simulink model "bh_SIM_7dof_car_VALIDATE"  (R2021a)
settings: Solver=ode15s  StartTime=0.0  StopTime=60  FixedStep=0.0005  RelTol=1e-5
libraries: simulink x1
settings Model: Creator=bhorton  LastModifiedBy=bhorton
settings SolverCC: ZeroCrossAlgorithm=Adaptive
settings ExplorerConfigSet: InternalSimMechanicsExplorerSettings="<ExplorerConfiguration><canonicalview>default</canonicalview><AnimationSetting><BasePlaybackSpeed>1.0</BasePlaybackSpeed><PlaybackSpeedFactor>1.0</PlaybackSpeedFactor></AnimationSetting><TilePanel><TileInfo><Tiles Columns=\"2\" Count=\"3\" Rows=\"2\"><Column Weight=\"0.4994\"/><Column Weight=\"0.5006\"/><Row Weight=\"0.4993\"/><Row Weight=\"0.5007\"/><Tile Height=\"1\" Width=\"2\" X=\"0\" Y=\"0\"/><Tile Height=\"1\" Width=\"1\" X=\"0\" Y=\"1\"/><Tile Height=\"1\" Width=\"1\" X=\"1\" Y=\"1\"/></Tiles></TileInfo><SceneInfo><SceneViewer><BGColor><R>0.60000002384185791</R><G>0.60000002384185791</G><B>0.60000002384185791</B></BGColor><Camera><DoPerspective>off</DoPerspective><Position><X>4.58629206826182401</X><Y>2.2090645401570459</Y><Z>2.36549759190957332</Z></Position><Center><X>2.57683900679416</X><Y>1.27770136551759128</Y><Z>-0.515230289296268573</Z></Center><Up><X>-0.185673330126828295</X><Y>0.96548958646651295</Y><Z>-0.182634259941381938</Z></Up><ViewLimDist>1</ViewLimDist><YLim>2.38220316698246792</YLim><XLim>4.86337026375055714</XLim></Camera></SceneViewer><SceneViewer><BGColor><R>0.60000002384185791</R><G>0.60000002384185791</G><B>0.60000002384185791</B></BGColor><Camera><DoPerspective>off</DoPerspective><Position><X>1.59253986433018846</X><Y>1.4781034625054259</Y><Z>2.45336125750569334</Z></Position><Center><X>1.41562813270534282</X><Y>1.03964723052633357</Y><Z>-0.792996094118513462</Z></Center><Up><X>-0.0228131350943184333</X><Y>0.990908416802929626</Y><Z>-0.132589857742894418</Z></Up><ViewLimDist>1</ViewLimDist><YLim>1.71081238252217549</YLim><XLim>1.71587395761839479</XLim></Camera></SceneViewer><SceneViewer><BGColor><R>0.60000002384185791</R><G>0.60000002384185791</G><B>0.60000002384185791</B></BGColor><Camera><DoPerspective>off</DoPerspective><Position><X>5.22556337212071131</X><Y>1.49802244333944778</Y><Z>-0.435936726178495881</Z></Position><Center><X>1.55561505094653896</X><Y>1.09424096945505833</Y><Z>-0.658674871233751014</Z></Center><Up><X>-0.109797444713875203</X><Y>0.993927323497863835</Y><Z>0.0072798858972461869</Z></Up><ViewLimDist>1</ViewLimDist><YLim>2.32163445502303123</YLim><XLim>2.33537193700541623</XLim></Camera></SceneViewer></SceneInfo></TilePanel><MechEditorPanel><Cameras/><GfxPanelCameraMap/><VideoCreator><PlaybackSpeedRatio>1.0</PlaybackSpeedRatio><FrameRate>30</FrameRate><VideoFormat>MPEG-4</VideoFormat><FrameSize>[800 600]</FrameSize></VideoCreator></MechEditorPanel></ExplorerConfiguration>"

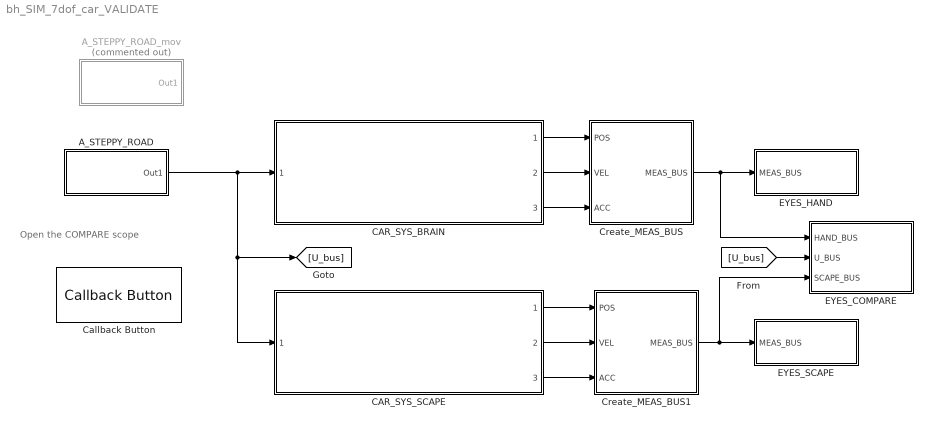
== system bh_SIM_7dof_car_VALIDATE ==
  note: Open the COMPARE scope
  A_STEPPY_ROAD : Subsystem
  A_STEPPY_ROAD_mov : Subsystem  Commented=on
  CAR_SYS_BRAIN : Subsystem  ReferencedSubsystem=bh_COMPONENT_model_7dof_car_HAND  L_b=OBJ_car_params.L_b  L_f=OBJ_car_params.L_f  L_R=OBJ_car_params.L_R  L_L=OBJ_car_params.L_L  m_c=OBJ_car_params.m_c  I_cZ=OBJ_car_params.I_cZ  I_cX=OBJ_car_params.I_cX  m_bR=OBJ_car_params.m_bR  m_fR=OBJ_car_params.m_fR  m_bL=OBJ_car_params.m_bL  m_fL=OBJ_car_params.m_fL  k_bR=OBJ_car_params.k_bR  k_fR=OBJ_car_params.k_fR  k_bL=OBJ_car_params.k_bL  k_fL=OBJ_car_params.k_fL  k_bRG=OBJ_car_params.k_bRG  k_fRG=OBJ_car_params.k_fRG  k_bLG=OBJ_car_params.k_bLG  k_fLG=OBJ_car_params.k_fLG  c_bR=OBJ_car_params.c_bR  c_fR=OBJ_car_params.c_fR  c_bL=OBJ_car_params.c_bL  c_fL=OBJ_car_params.c_fL  c_bRG=OBJ_car_params.c_bRG  c_fRG=OBJ_car_params.c_fRG  c_bLG=OBJ_car_params.c_bLG  c_fLG=OBJ_car_params.c_fLG  IC_pos=OBJ_car_params.IC_pos  IC_vel=OBJ_car_params.IC_vel
  CAR_SYS_SCAPE : Subsystem  ReferencedSubsystem=bh_COMPONENT_model_7dof_car_SCAPE  L_b=OBJ_car_params.L_b  L_f=OBJ_car_params.L_f  L_R=OBJ_car_params.L_R  L_L=OBJ_car_params.L_L  m_c=OBJ_car_params.m_c  I_cZ=OBJ_car_params.I_cZ  I_cX=OBJ_car_params.I_cX  m_bR=OBJ_car_params.m_bR  m_fR=OBJ_car_params.m_fR  m_bL=OBJ_car_params.m_bL  m_fL=OBJ_car_params.m_fL  k_bR=OBJ_car_params.k_bR  k_fR=OBJ_car_params.k_fR  k_bL=OBJ_car_params.k_bL  k_fL=OBJ_car_params.k_fL  k_bRG=OBJ_car_params.k_bRG  k_fRG=OBJ_car_params.k_fRG  k_bLG=OBJ_car_params.k_bLG  k_fLG=OBJ_car_params.k_fLG  c_bR=OBJ_car_params.c_bR  c_fR=OBJ_car_params.c_fR  c_bL=OBJ_car_params.c_bL  c_fL=OBJ_car_params.c_fL  c_bRG=OBJ_car_params.c_bRG  c_fRG=OBJ_car_params.c_fRG  c_bLG=OBJ_car_params.c_bLG  c_fLG=OBJ_car_params.c_fLG  IC_pos=OBJ_car_params.IC_pos  IC_vel=OBJ_car_params.IC_vel
  Callback Button : CallbackButton  ButtonText=CLICK me to open SCOPE
      settings: ClickFcn=open_system([bdroot,'/EYES_COMPARE/COMPARE_POS'])
  Create_MEAS_BUS : Subsystem
  Create_MEAS_BUS1 : Subsystem
  EYES_COMPARE : Subsystem
  EYES_HAND : Subsystem
  EYES_SCAPE : Subsystem
  wires:
  CAR_SYS_BRAIN/1 -> Create_MEAS_BUS/1(POS)
  CAR_SYS_BRAIN/2 -> Create_MEAS_BUS/2(VEL)
  CAR_SYS_BRAIN/3 -> Create_MEAS_BUS/3(ACC)
  Create_MEAS_BUS/1(MEAS_BUS) -> EYES_COMPARE/1(HAND_BUS), EYES_HAND/1(MEAS_BUS)
  CAR_SYS_SCAPE/1 -> Create_MEAS_BUS1/1(POS)
  CAR_SYS_SCAPE/2 -> Create_MEAS_BUS1/2(VEL)
  CAR_SYS_SCAPE/3 -> Create_MEAS_BUS1/3(ACC)
  Create_MEAS_BUS1/1(MEAS_BUS) -> EYES_COMPARE/3(SCAPE_BUS), EYES_SCAPE/1(MEAS_BUS)
  A_STEPPY_ROAD/1(Out1) -> [U_bus], CAR_SYS_SCAPE/1, CAR_SYS_BRAIN/1
  [U_bus] -> EYES_COMPARE/2(U_BUS)

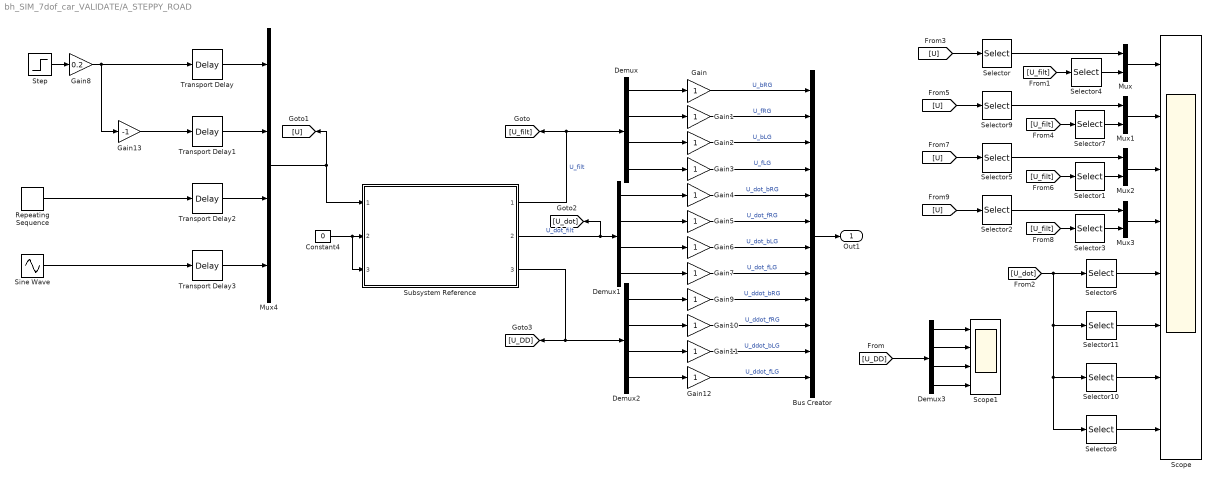
== system bh_SIM_7dof_car_VALIDATE/A_STEPPY_ROAD ==
  Bus Creator : BusCreator  Inputs=12
  Constant4 : Constant  Value=0
  Demux{,1..3} (4 alike) : Demux
  Gain{,1..7,9..12} (12 alike) : Gain
  Gain13 : Gain  Gain=-1
  Gain8 : Gain  Gain=0.2
  Mux{,1..3} (4 alike) : Mux  Inputs=2
  Mux4 : Mux
  Repeating Sequence : simulink/Sources/Repeating Sequence  rep_seq_t=[0 2]  rep_seq_y=[0 0.2]
  Scope : Scope  NumInputPorts=8
  Scope1 : Scope  NumInputPorts=4
  Selector : Selector  InputPortWidth=4  IndexOptions=Index vector (dialog)  Indices=1  OutputSizes=1
  Selector1 : Selector  InputPortWidth=4  IndexOptions=Index vector (dialog)  Indices=3  OutputSizes=1
  Selector10 : Selector  InputPortWidth=4  IndexOptions=Index vector (dialog)  Indices=3  OutputSizes=1
  Selector11 : Selector  InputPortWidth=4  IndexOptions=Index vector (dialog)  Indices=2  OutputSizes=1
  Selector2 : Selector  InputPortWidth=4  IndexOptions=Index vector (dialog)  Indices=4  OutputSizes=1
  Selector3 : Selector  InputPortWidth=4  IndexOptions=Index vector (dialog)  Indices=4  OutputSizes=1
  Selector4 : Selector  InputPortWidth=4  IndexOptions=Index vector (dialog)  Indices=1  OutputSizes=1
  Selector5 : Selector  InputPortWidth=4  IndexOptions=Index vector (dialog)  Indices=3  OutputSizes=1
  Selector6 : Selector  InputPortWidth=4  IndexOptions=Index vector (dialog)  Indices=1  OutputSizes=1
  Selector7 : Selector  InputPortWidth=4  IndexOptions=Index vector (dialog)  Indices=2  OutputSizes=1
  Selector8 : Selector  InputPortWidth=4  IndexOptions=Index vector (dialog)  Indices=4  OutputSizes=1
  Selector9 : Selector  InputPortWidth=4  IndexOptions=Index vector (dialog)  Indices=2  OutputSizes=1
  Sine Wave : Sin  Amplitude=0.25  Frequency=2*pi*3  SampleTime=0
  Step : Step  Time=0  SampleTime=0
  Subsystem Reference : Subsystem  ReferencedSubsystem=bh_COMPONENT_deriv_est  wn=2*pi*5000  p=1
  Transport Delay : TransportDelay  DelayTime=20
      settings: AttributesFormatString=Delay =%<DelayTime> (secs)
  Transport Delay1 : TransportDelay  DelayTime=30
      settings: AttributesFormatString=Delay =%<DelayTime> (secs)
  Transport Delay2 : TransportDelay  DelayTime=40
      settings: AttributesFormatString=Delay =%<DelayTime> (secs)
  Transport Delay3 : TransportDelay  DelayTime=50
      settings: AttributesFormatString=Delay =%<DelayTime> (secs)
  Out1 : Outport
  wires:
  Selector8/1 -> Scope/8
  Subsystem Reference/3 -> [U_DD], Demux2/1
  Demux2/4 -> Gain12/1
  Demux/3 -> Gain2/1
  Selector1/1 -> Mux2/2
  Gain5/1 -> Bus Creator/6  "U_dot_fRG"
  Subsystem Reference/1 -> [U_filt], Demux/1  "U_filt"
  Gain6/1 -> Bus Creator/7  "U_dot_bLG"
  Gain7/1 -> Bus Creator/8  "U_dot_fLG"
  Gain11/1 -> Bus Creator/11  "U_ddot_bLG"
  Subsystem Reference/2 -> [U_dot], Demux1/1  "U_dot_filt"
  Constant4/1 -> Subsystem Reference/3, Subsystem Reference/2
  [U_DD] -> Demux3/1
  Demux3/3 -> Scope1/3
  Demux3/2 -> Scope1/2
  Gain/1 -> Bus Creator/1  "U_bRG"
  Demux2/2 -> Gain10/1
  Selector2/1 -> Mux3/1
  Gain12/1 -> Bus Creator/12  "U_ddot_fLG"
  Gain9/1 -> Bus Creator/9  "U_ddot_bRG"
  Gain10/1 -> Bus Creator/10  "U_ddot_fRG"
  Mux1/1 -> Scope/2
  [U_filt] -> Selector3/1
  Selector6/1 -> Scope/5
  Demux3/4 -> Scope1/4
  Selector5/1 -> Mux2/1
  Demux2/3 -> Gain11/1
  Demux2/1 -> Gain9/1
  Mux2/1 -> Scope/3
  Demux3/1 -> Scope1/1
  Selector/1 -> Mux/1
  [U] -> Selector2/1
  Bus Creator/1 -> Out1/1
  Selector3/1 -> Mux3/2
  Selector7/1 -> Mux1/2
  Demux1/4 -> Gain7/1
  [U] -> Selector9/1
  Selector9/1 -> Mux1/1
  Mux3/1 -> Scope/4
  [U] -> Selector/1
  Selector4/1 -> Mux/2
  Mux/1 -> Scope/1
  [U_filt] -> Selector1/1
  [U] -> Selector5/1
  Demux1/3 -> Gain6/1
  Demux/2 -> Gain1/1
  [U_dot] -> Selector11/1, Selector10/1, Selector8/1, Selector6/1
  Demux/1 -> Gain/1
  Gain4/1 -> Bus Creator/5  "U_dot_bRG"
  [U_filt] -> Selector7/1
  [U_filt] -> Selector4/1
  Demux1/2 -> Gain5/1
  Gain3/1 -> Bus Creator/4  "U_fLG"
  Selector10/1 -> Scope/7
  Selector11/1 -> Scope/6
  Demux/4 -> Gain3/1
  Gain1/1 -> Bus Creator/2  "U_fRG"
  Demux1/1 -> Gain4/1
  Gain2/1 -> Bus Creator/3  "U_bLG"
  Mux4/1 -> Subsystem Reference/1, [U]
  Step/1 -> Gain8/1
  Transport Delay/1 -> Mux4/1
  Transport Delay1/1 -> Mux4/2
  Transport Delay2/1 -> Mux4/3
  Transport Delay3/1 -> Mux4/4
  Gain8/1 -> Gain13/1, Transport Delay/1
  Sine Wave/1 -> Transport Delay3/1
  Gain13/1 -> Transport Delay1/1
  Repeating Sequence/1 -> Transport Delay2/1

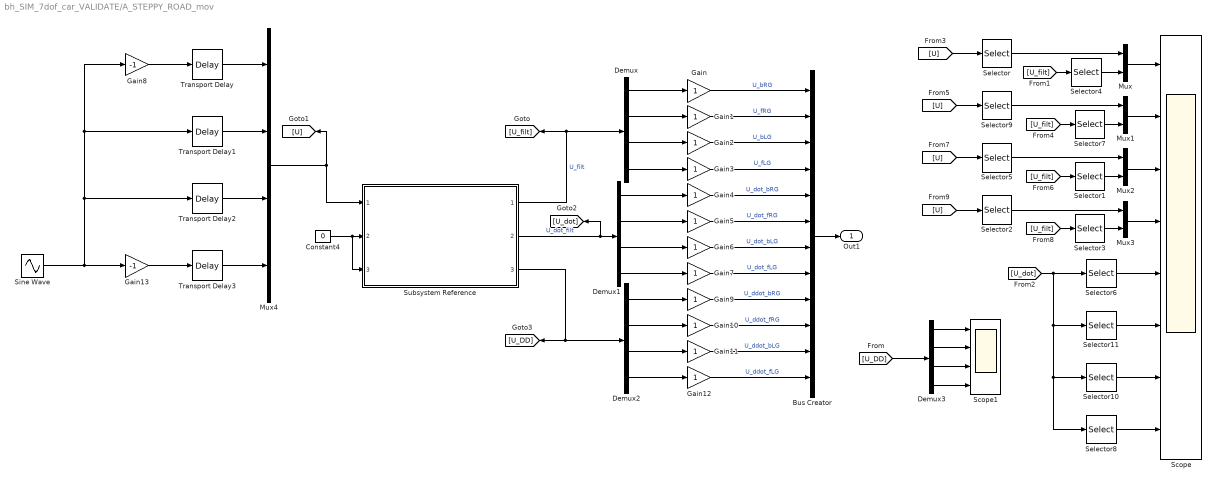
== system bh_SIM_7dof_car_VALIDATE/A_STEPPY_ROAD_mov ==
  Bus Creator : BusCreator  Inputs=12
  Constant4 : Constant  Value=0
  Demux{,1..3} (4 alike) : Demux
  Gain{,1..7,9..12} (12 alike) : Gain
  Gain13 : Gain  Gain=-1
  Gain8 : Gain  Gain=-1
  Mux{,1..3} (4 alike) : Mux  Inputs=2
  Mux4 : Mux
  Scope : Scope  NumInputPorts=8
  Scope1 : Scope  NumInputPorts=4
  Selector : Selector  InputPortWidth=4  IndexOptions=Index vector (dialog)  Indices=1  OutputSizes=1
  Selector1 : Selector  InputPortWidth=4  IndexOptions=Index vector (dialog)  Indices=3  OutputSizes=1
  Selector10 : Selector  InputPortWidth=4  IndexOptions=Index vector (dialog)  Indices=3  OutputSizes=1
  Selector11 : Selector  InputPortWidth=4  IndexOptions=Index vector (dialog)  Indices=2  OutputSizes=1
  Selector2 : Selector  InputPortWidth=4  IndexOptions=Index vector (dialog)  Indices=4  OutputSizes=1
  Selector3 : Selector  InputPortWidth=4  IndexOptions=Index vector (dialog)  Indices=4  OutputSizes=1
  Selector4 : Selector  InputPortWidth=4  IndexOptions=Index vector (dialog)  Indices=1  OutputSizes=1
  Selector5 : Selector  InputPortWidth=4  IndexOptions=Index vector (dialog)  Indices=3  OutputSizes=1
  Selector6 : Selector  InputPortWidth=4  IndexOptions=Index vector (dialog)  Indices=1  OutputSizes=1
  Selector7 : Selector  InputPortWidth=4  IndexOptions=Index vector (dialog)  Indices=2  OutputSizes=1
  Selector8 : Selector  InputPortWidth=4  IndexOptions=Index vector (dialog)  Indices=4  OutputSizes=1
  Selector9 : Selector  InputPortWidth=4  IndexOptions=Index vector (dialog)  Indices=2  OutputSizes=1
  Sine Wave : Sin  Amplitude=0.15  Frequency=2*pi*2  SampleTime=0
  Subsystem Reference : Subsystem  ReferencedSubsystem=bh_COMPONENT_deriv_est  wn=2*pi*5000  p=1
  Transport Delay{,1..3} (4 alike) : TransportDelay  DelayTime=10
      settings: AttributesFormatString=Delay =%<DelayTime> (secs)
  Out1 : Outport
  wires:
  Selector8/1 -> Scope/8
  Subsystem Reference/3 -> [U_DD], Demux2/1
  Demux2/4 -> Gain12/1
  Demux/3 -> Gain2/1
  Selector1/1 -> Mux2/2
  Gain5/1 -> Bus Creator/6  "U_dot_fRG"
  Subsystem Reference/1 -> [U_filt], Demux/1  "U_filt"
  Gain6/1 -> Bus Creator/7  "U_dot_bLG"
  Gain7/1 -> Bus Creator/8  "U_dot_fLG"
  Gain11/1 -> Bus Creator/11  "U_ddot_bLG"
  Subsystem Reference/2 -> [U_dot], Demux1/1  "U_dot_filt"
  Constant4/1 -> Subsystem Reference/3, Subsystem Reference/2
  [U_DD] -> Demux3/1
  Demux3/3 -> Scope1/3
  Demux3/2 -> Scope1/2
  Gain/1 -> Bus Creator/1  "U_bRG"
  Demux2/2 -> Gain10/1
  Selector2/1 -> Mux3/1
  Gain12/1 -> Bus Creator/12  "U_ddot_fLG"
  Gain9/1 -> Bus Creator/9  "U_ddot_bRG"
  Gain10/1 -> Bus Creator/10  "U_ddot_fRG"
  Mux1/1 -> Scope/2
  [U_filt] -> Selector3/1
  Selector6/1 -> Scope/5
  Demux3/4 -> Scope1/4
  Selector5/1 -> Mux2/1
  Demux2/3 -> Gain11/1
  Demux2/1 -> Gain9/1
  Mux2/1 -> Scope/3
  Demux3/1 -> Scope1/1
  Selector/1 -> Mux/1
  [U] -> Selector2/1
  Bus Creator/1 -> Out1/1
  Selector3/1 -> Mux3/2
  Selector7/1 -> Mux1/2
  Demux1/4 -> Gain7/1
  [U] -> Selector9/1
  Selector9/1 -> Mux1/1
  Mux3/1 -> Scope/4
  [U] -> Selector/1
  Selector4/1 -> Mux/2
  Mux/1 -> Scope/1
  [U_filt] -> Selector1/1
  [U] -> Selector5/1
  Demux1/3 -> Gain6/1
  Demux/2 -> Gain1/1
  [U_dot] -> Selector11/1, Selector10/1, Selector8/1, Selector6/1
  Demux/1 -> Gain/1
  Gain4/1 -> Bus Creator/5  "U_dot_bRG"
  [U_filt] -> Selector7/1
  [U_filt] -> Selector4/1
  Demux1/2 -> Gain5/1
  Gain3/1 -> Bus Creator/4  "U_fLG"
  Selector10/1 -> Scope/7
  Selector11/1 -> Scope/6
  Demux/4 -> Gain3/1
  Gain1/1 -> Bus Creator/2  "U_fRG"
  Demux1/1 -> Gain4/1
  Gain2/1 -> Bus Creator/3  "U_bLG"
  Mux4/1 -> Subsystem Reference/1, [U]
  Transport Delay/1 -> Mux4/1
  Transport Delay1/1 -> Mux4/2
  Transport Delay2/1 -> Mux4/3
  Transport Delay3/1 -> Mux4/4
  Sine Wave/1 -> Transport Delay2/1, Transport Delay1/1, Gain8/1, Gain13/1
  Gain8/1 -> Transport Delay/1
  Gain13/1 -> Transport Delay3/1

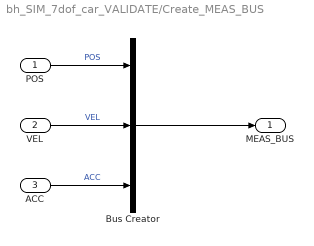
== system bh_SIM_7dof_car_VALIDATE/Create_MEAS_BUS ==
  POS : Inport
  VEL : Inport  Port=2
  ACC : Inport  Port=3
  Bus Creator : BusCreator  Inputs=3
  MEAS_BUS : Outport
  wires:
  POS/1 -> Bus Creator/1  "POS"
  VEL/1 -> Bus Creator/2  "VEL"
  ACC/1 -> Bus Creator/3  "ACC"
  Bus Creator/1 -> MEAS_BUS/1

== system bh_SIM_7dof_car_VALIDATE/Create_MEAS_BUS1 ==
  POS : Inport
  VEL : Inport  Port=2
  ACC : Inport  Port=3
  Bus Creator : BusCreator  Inputs=3
  MEAS_BUS : Outport
  wires:
  POS/1 -> Bus Creator/1  "POS"
  VEL/1 -> Bus Creator/2  "VEL"
  ACC/1 -> Bus Creator/3  "ACC"
  Bus Creator/1 -> MEAS_BUS/1

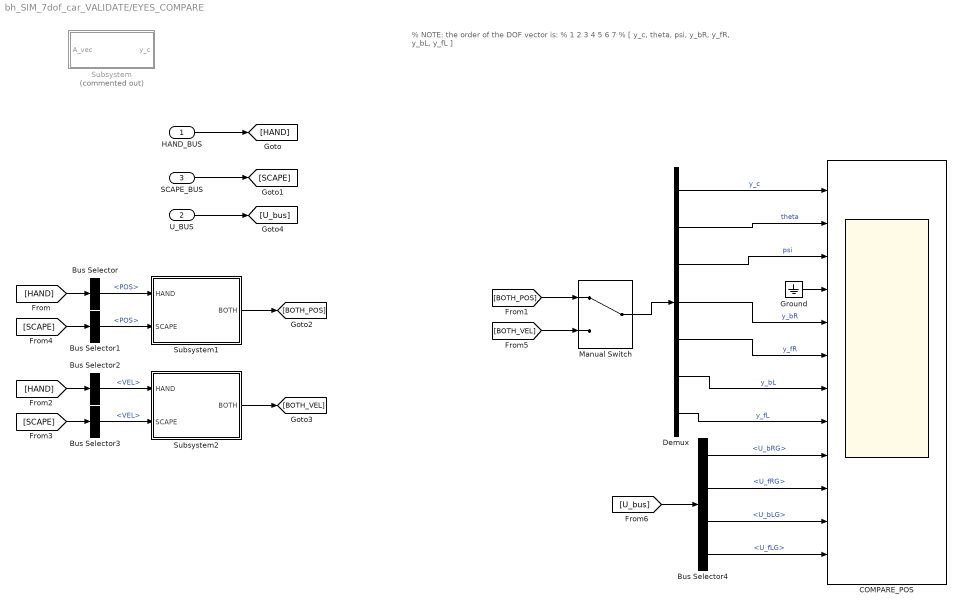
== system bh_SIM_7dof_car_VALIDATE/EYES_COMPARE ==
  note: % NOTE:  the order of the DOF vector is:
      | %          1      2    3     4     5     6     7
      | %      [ y_c, theta, psi, y_bR, y_fR, y_bL, y_fL ]
  HAND_BUS : Inport
  U_BUS : Inport  Port=2
  SCAPE_BUS : Inport  Port=3
  Bus Selector : BusSelector  OutputSignals=POS
  Bus Selector1 : BusSelector  OutputSignals=POS
  Bus Selector2 : BusSelector  OutputSignals=VEL
  Bus Selector3 : BusSelector  OutputSignals=VEL
  Bus Selector4 : BusSelector  OutputSignals=U_bRG,U_fRG,U_bLG,U_fLG
  COMPARE_POS : Scope  NumInputPorts=12
  Demux : Demux  Outputs=7
  Ground : Ground
  Manual Switch : ManualSwitch
  Subsystem : Subsystem  Commented=on
  Subsystem1 : Subsystem
  Subsystem2 : Subsystem
  wires:
  HAND_BUS/1 -> [HAND]
  Demux/1 -> COMPARE_POS/1  "y_c"
  Demux/2 -> COMPARE_POS/2  "theta"
  Demux/3 -> COMPARE_POS/3  "psi"
  Ground/1 -> COMPARE_POS/4
  Demux/5 -> COMPARE_POS/6  "y_fR"
  Demux/6 -> COMPARE_POS/7  "y_bL"
  Demux/7 -> COMPARE_POS/8  "y_fL"
  SCAPE_BUS/1 -> [SCAPE]
  [HAND] -> Bus Selector/1
  [SCAPE] -> Bus Selector1/1
  Bus Selector/1 -> Subsystem1/1(HAND)  "<POS>"
  Bus Selector1/1 -> Subsystem1/2(SCAPE)  "<POS>"
  Subsystem1/1(BOTH) -> [BOTH_POS]
  [HAND] -> Bus Selector2/1
  Subsystem2/1(BOTH) -> [BOTH_VEL]
  Bus Selector2/1 -> Subsystem2/1(HAND)  "<VEL>"
  Bus Selector3/1 -> Subsystem2/2(SCAPE)  "<VEL>"
  [SCAPE] -> Bus Selector3/1
  Manual Switch/1 -> Demux/1
  [BOTH_VEL] -> Manual Switch/2
  [BOTH_POS] -> Manual Switch/1
  U_BUS/1 -> [U_bus]
  [U_bus] -> Bus Selector4/1
  Bus Selector4/4 -> COMPARE_POS/12  "<U_fLG>"
  Bus Selector4/3 -> COMPARE_POS/11  "<U_bLG>"
  Bus Selector4/2 -> COMPARE_POS/10  "<U_fRG>"
  Bus Selector4/1 -> COMPARE_POS/9  "<U_bRG>"
  Demux/4 -> COMPARE_POS/5  "y_bR"

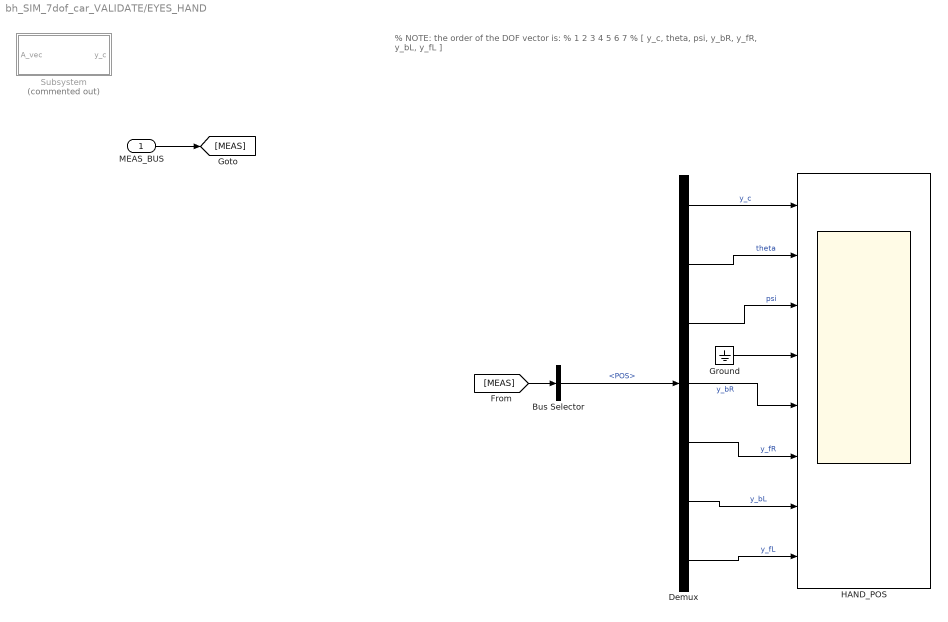
== system bh_SIM_7dof_car_VALIDATE/EYES_HAND ==
  note: % NOTE:  the order of the DOF vector is:
      | %          1      2    3     4     5     6     7
      | %      [ y_c, theta, psi, y_bR, y_fR, y_bL, y_fL ]
  MEAS_BUS : Inport
  Bus Selector : BusSelector  OutputSignals=POS
  Demux : Demux  Outputs=7
  Ground : Ground
  HAND_POS : Scope  NumInputPorts=8
  Subsystem : Subsystem  Commented=on
  wires:
  MEAS_BUS/1 -> [MEAS]
  Demux/1 -> HAND_POS/1  "y_c"
  Demux/2 -> HAND_POS/2  "theta"
  Demux/3 -> HAND_POS/3  "psi"
  Ground/1 -> HAND_POS/4
  Demux/4 -> HAND_POS/5  "y_bR"
  Demux/5 -> HAND_POS/6  "y_fR"
  Demux/6 -> HAND_POS/7  "y_bL"
  Demux/7 -> HAND_POS/8  "y_fL"
  [MEAS] -> Bus Selector/1
  Bus Selector/1 -> Demux/1  "<POS>"

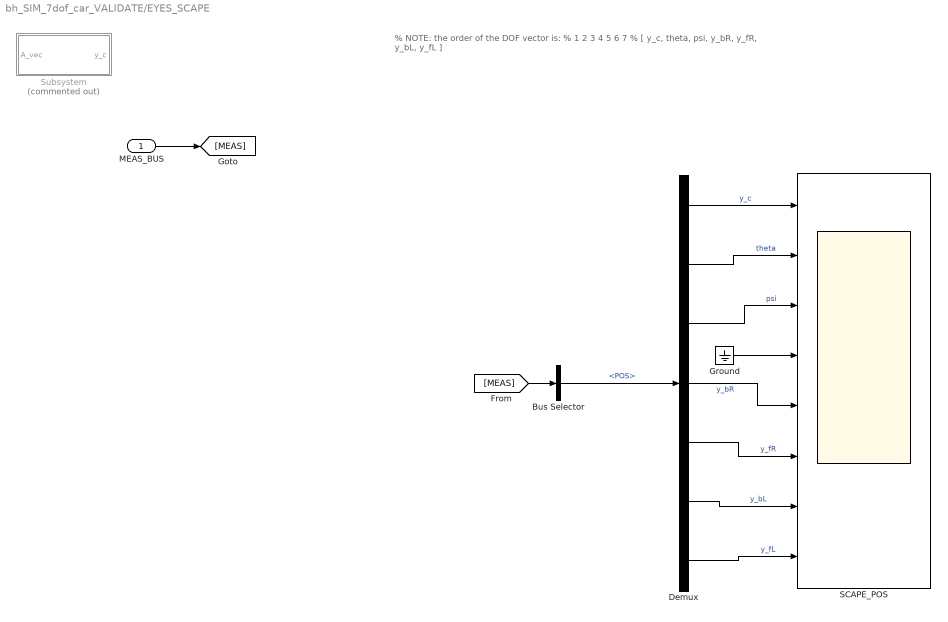
== system bh_SIM_7dof_car_VALIDATE/EYES_SCAPE ==
  note: % NOTE:  the order of the DOF vector is:
      | %          1      2    3     4     5     6     7
      | %      [ y_c, theta, psi, y_bR, y_fR, y_bL, y_fL ]
  MEAS_BUS : Inport
  Bus Selector : BusSelector  OutputSignals=POS
  Demux : Demux  Outputs=7
  Ground : Ground
  SCAPE_POS : Scope  NumInputPorts=8
  Subsystem : Subsystem  Commented=on
  wires:
  MEAS_BUS/1 -> [MEAS]
  Demux/1 -> SCAPE_POS/1  "y_c"
  Demux/2 -> SCAPE_POS/2  "theta"
  Demux/3 -> SCAPE_POS/3  "psi"
  Ground/1 -> SCAPE_POS/4
  Demux/4 -> SCAPE_POS/5  "y_bR"
  Demux/5 -> SCAPE_POS/6  "y_fR"
  Demux/6 -> SCAPE_POS/7  "y_bL"
  Demux/7 -> SCAPE_POS/8  "y_fL"
  [MEAS] -> Bus Selector/1
  Bus Selector/1 -> Demux/1  "<POS>"

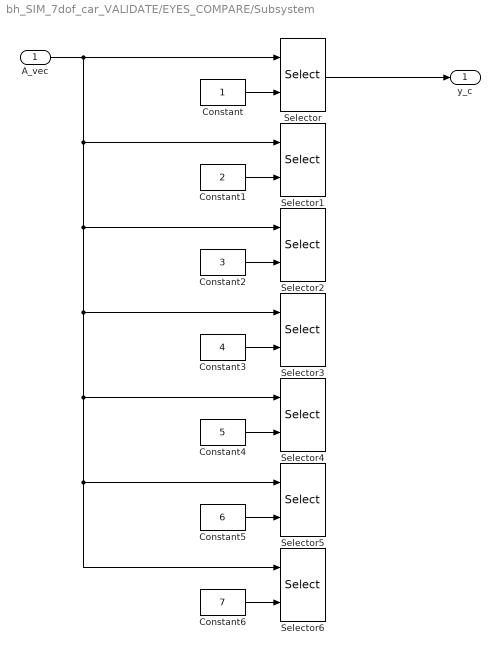
== system bh_SIM_7dof_car_VALIDATE/EYES_COMPARE/Subsystem ==
  A_vec : Inport
  Constant : Constant
  Constant1 : Constant  Value=2
  Constant2 : Constant  Value=3
  Constant3 : Constant  Value=4
  Constant4 : Constant  Value=5
  Constant5 : Constant  Value=6
  Constant6 : Constant  Value=7
  Selector{,1..6} (7 alike) : Selector  InputPortWidth=7  IndexOptions=Index vector (port)  Indices=1  OutputSizes=1
  y_c : Outport
  wires:
  Constant/1 -> Selector/2
  Constant1/1 -> Selector1/2
  Constant2/1 -> Selector2/2
  Constant3/1 -> Selector3/2
  Constant4/1 -> Selector4/2
  Constant5/1 -> Selector5/2
  Constant6/1 -> Selector6/2
  A_vec/1 -> Selector1/1, Selector2/1, Selector3/1, Selector4/1, Selector5/1, Selector6/1, Selector/1
  Selector/1 -> y_c/1

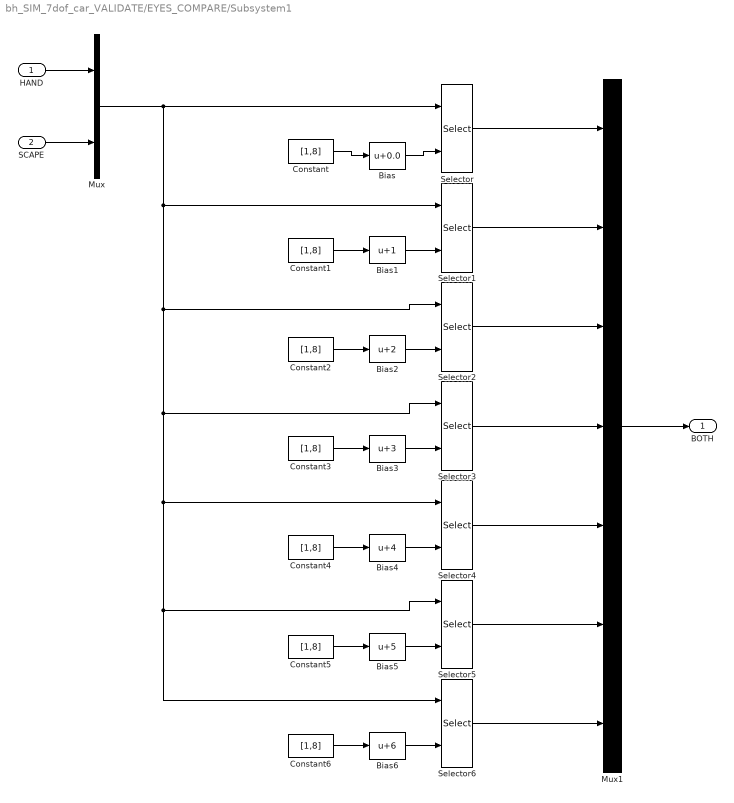
== system bh_SIM_7dof_car_VALIDATE/EYES_COMPARE/Subsystem1 ==
  HAND : Inport
  SCAPE : Inport  Port=2
  Bias : Bias  Bias=0.0
  Bias1 : Bias  Bias=1
  Bias2 : Bias  Bias=2
  Bias3 : Bias  Bias=3
  Bias4 : Bias  Bias=4
  Bias5 : Bias  Bias=5
  Bias6 : Bias  Bias=6
  Constant{,1..6} (7 alike) : Constant  Value=[1,8]
  Mux : Mux  Inputs=2
  Mux1 : Mux  Inputs=7
  Selector{,1..6} (7 alike) : Selector  InputPortWidth=14  IndexOptions=Index vector (port)  Indices=[1 3]  OutputSizes=1
  BOTH : Outport
  wires:
  SCAPE/1 -> Mux/2
  HAND/1 -> Mux/1
  Constant/1 -> Bias/1
  Bias/1 -> Selector/2
  Selector/1 -> Mux1/1
  Selector1/1 -> Mux1/2
  Bias1/1 -> Selector1/2
  Constant1/1 -> Bias1/1
  Constant2/1 -> Bias2/1
  Bias2/1 -> Selector2/2
  Selector2/1 -> Mux1/3
  Bias3/1 -> Selector3/2
  Constant3/1 -> Bias3/1
  Selector3/1 -> Mux1/4
  Constant4/1 -> Bias4/1
  Bias4/1 -> Selector4/2
  Selector4/1 -> Mux1/5
  Constant5/1 -> Bias5/1
  Bias5/1 -> Selector5/2
  Constant6/1 -> Bias6/1
  Bias6/1 -> Selector6/2
  Mux/1 -> Selector1/1, Selector2/1, Selector3/1, Selector4/1, Selector5/1, Selector6/1, Selector/1
  Selector5/1 -> Mux1/6
  Selector6/1 -> Mux1/7
  Mux1/1 -> BOTH/1

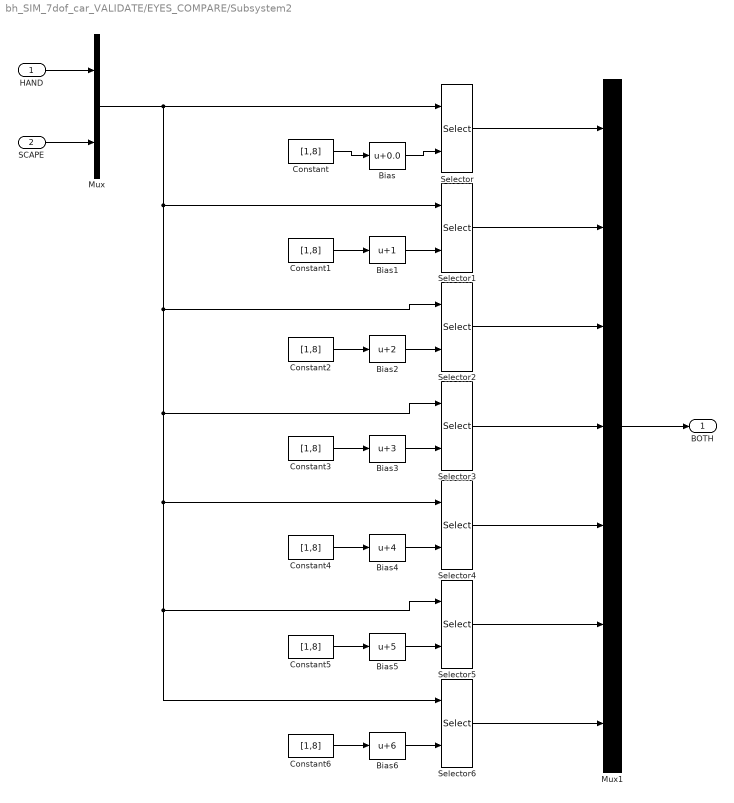
== system bh_SIM_7dof_car_VALIDATE/EYES_COMPARE/Subsystem2 ==
  HAND : Inport
  SCAPE : Inport  Port=2
  Bias : Bias  Bias=0.0
  Bias1 : Bias  Bias=1
  Bias2 : Bias  Bias=2
  Bias3 : Bias  Bias=3
  Bias4 : Bias  Bias=4
  Bias5 : Bias  Bias=5
  Bias6 : Bias  Bias=6
  Constant{,1..6} (7 alike) : Constant  Value=[1,8]
  Mux : Mux  Inputs=2
  Mux1 : Mux  Inputs=7
  Selector{,1..6} (7 alike) : Selector  InputPortWidth=14  IndexOptions=Index vector (port)  Indices=[1 3]  OutputSizes=1
  BOTH : Outport
  wires:
  SCAPE/1 -> Mux/2
  HAND/1 -> Mux/1
  Constant/1 -> Bias/1
  Bias/1 -> Selector/2
  Selector/1 -> Mux1/1
  Selector1/1 -> Mux1/2
  Bias1/1 -> Selector1/2
  Constant1/1 -> Bias1/1
  Constant2/1 -> Bias2/1
  Bias2/1 -> Selector2/2
  Selector2/1 -> Mux1/3
  Bias3/1 -> Selector3/2
  Constant3/1 -> Bias3/1
  Selector3/1 -> Mux1/4
  Constant4/1 -> Bias4/1
  Bias4/1 -> Selector4/2
  Selector4/1 -> Mux1/5
  Constant5/1 -> Bias5/1
  Bias5/1 -> Selector5/2
  Constant6/1 -> Bias6/1
  Bias6/1 -> Selector6/2
  Mux/1 -> Selector1/1, Selector2/1, Selector3/1, Selector4/1, Selector5/1, Selector6/1, Selector/1
  Selector5/1 -> Mux1/6
  Selector6/1 -> Mux1/7
  Mux1/1 -> BOTH/1

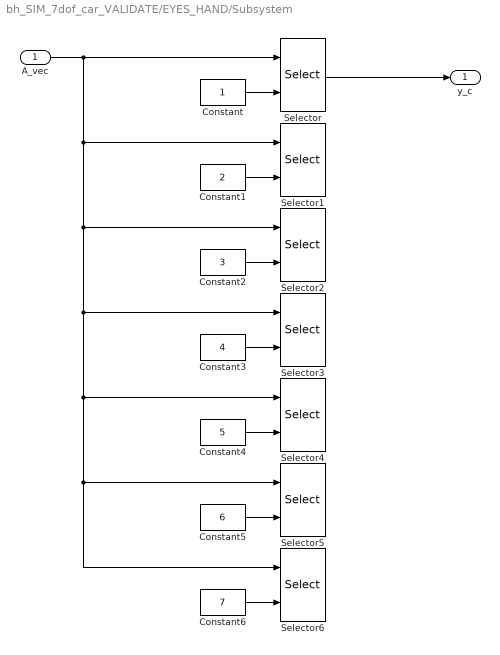
== system bh_SIM_7dof_car_VALIDATE/EYES_HAND/Subsystem ==
  A_vec : Inport
  Constant : Constant
  Constant1 : Constant  Value=2
  Constant2 : Constant  Value=3
  Constant3 : Constant  Value=4
  Constant4 : Constant  Value=5
  Constant5 : Constant  Value=6
  Constant6 : Constant  Value=7
  Selector{,1..6} (7 alike) : Selector  InputPortWidth=7  IndexOptions=Index vector (port)  Indices=1  OutputSizes=1
  y_c : Outport
  wires:
  Constant/1 -> Selector/2
  Constant1/1 -> Selector1/2
  Constant2/1 -> Selector2/2
  Constant3/1 -> Selector3/2
  Constant4/1 -> Selector4/2
  Constant5/1 -> Selector5/2
  Constant6/1 -> Selector6/2
  A_vec/1 -> Selector1/1, Selector2/1, Selector3/1, Selector4/1, Selector5/1, Selector6/1, Selector/1
  Selector/1 -> y_c/1

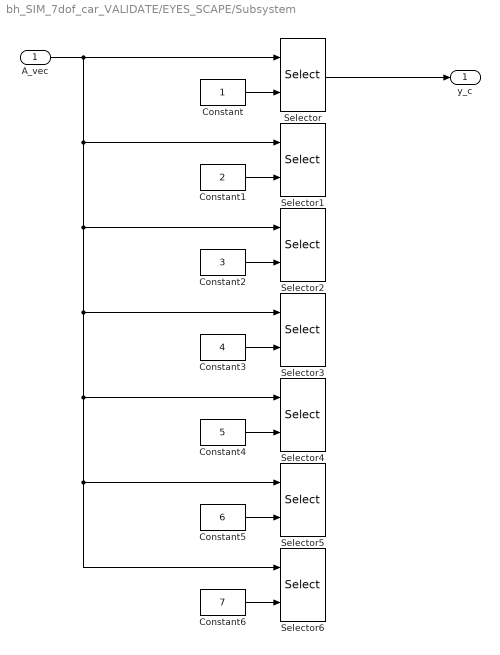
== system bh_SIM_7dof_car_VALIDATE/EYES_SCAPE/Subsystem ==
  A_vec : Inport
  Constant : Constant
  Constant1 : Constant  Value=2
  Constant2 : Constant  Value=3
  Constant3 : Constant  Value=4
  Constant4 : Constant  Value=5
  Constant5 : Constant  Value=6
  Constant6 : Constant  Value=7
  Selector{,1..6} (7 alike) : Selector  InputPortWidth=7  IndexOptions=Index vector (port)  Indices=1  OutputSizes=1
  y_c : Outport
  wires:
  Constant/1 -> Selector/2
  Constant1/1 -> Selector1/2
  Constant2/1 -> Selector2/2
  Constant3/1 -> Selector3/2
  Constant4/1 -> Selector4/2
  Constant5/1 -> Selector5/2
  Constant6/1 -> Selector6/2
  A_vec/1 -> Selector1/1, Selector2/1, Selector3/1, Selector4/1, Selector5/1, Selector6/1, Selector/1
  Selector/1 -> y_c/1
